simulink model "motor_bihuan_PI_tiaosu1205"  (Simulink 7.3)
settings: Solver=ode23tb  StartTime=0.0  StopTime=5  RelTol=1e-3
libraries: powerlib x12, powerlib_extras x2
settings Model: Creator=Administrator  LastModifiedBy=Administrator

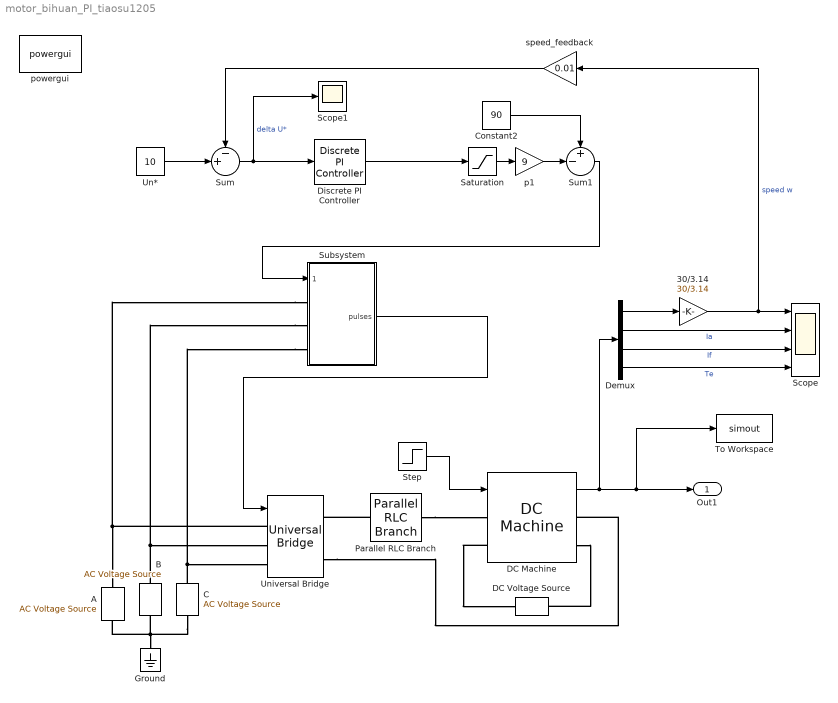
== system motor_bihuan_PI_tiaosu1205 ==
  30/3.14 : Gain  Gain=30/3.14  ParameterDataType=fixdt(1, 16)  ParameterScaling=2^0  OutDataType=fixdt(1, 16)  OutScaling=2^0
  A : powerlib/Electrical Sources/AC Voltage Source  DialogController=POWERSYS.PowerSysDialog  SystemSampleTime=-1  Amplitude=220  Phase=0  Frequency=50  SampleTime=0  Measurements=Voltage
  B : powerlib/Electrical Sources/AC Voltage Source  DialogController=POWERSYS.PowerSysDialog  SystemSampleTime=-1  Amplitude=220  Phase=240  Frequency=50  SampleTime=0  Measurements=Voltage
  C : powerlib/Electrical Sources/AC Voltage Source  DialogController=POWERSYS.PowerSysDialog  SystemSampleTime=-1  Amplitude=220  Phase=120  Frequency=50  SampleTime=0  Measurements=Voltage
  Constant2 : Constant  Value=90  OutDataType=fixdt(1, 16)  OutScaling=2^0
  DC Machine : powerlib/Machines/DC Machine  DialogController=POWERSYS.PowerSysDialog  SystemSampleTime=-1  PresetModel=No  MechanicalLoad=Torque TL  ShowDetailedParameters=on  RLa=[0.6 0.012]  RLf=[240 120]  Laf=1.8  J=1  Bm=0  Tf=0  w0=0  Ifinit=0.916666666666667  TsPowergui=0  TsBlock=-1
  DC Voltage Source : powerlib/Electrical Sources/DC Voltage Source  DialogController=POWERSYS.PowerSysDialog  SystemSampleTime=-1  Amplitude=220  Measurements=None
  Demux : Demux
  Discrete PI Controller : powerlib_extras/Discrete  Control Blocks/Discrete PI Controller  DialogController=POWERSYS.PowerSysDialog  SystemSampleTime=-1  Kp=1.2  Ki=2  Par_Limits=[1e6 -1e6]  Init=0  Ts=50e-6
  Ground : powerlib/Elements/Ground  DialogController=POWERSYS.PowerSysDialog  PhysicalDomain=powersysdomain  SubClassName=unknown  LeftPortType=p1  RightPortType=p1  LConnTagsString=a
  Parallel RLC Branch : powerlib/Elements/Parallel RLC Branch  DialogController=POWERSYS.PowerSysDialog  PhysicalDomain=powersysdomain  SubClassName=unknown  LeftPortType=p1  RightPortType=p1  LConnTagsString=a  RConnTagsString=__new0  BranchType=L  Resistance=1  Inductance=1e-3  SetiL0=off  InitialCurrent=0  Capacitance=1e-6  Setx0=off  InitialVoltage=0  Measurements=Branch voltage and current
  Saturation : Saturate  UpperLimit=10  LowerLimit=-10  OutDataType=fixdt(1, 16)  OutScaling=2^0
  Scope : Scope  NumInputPorts=4
      settings: TimeRange=5  YMin=-250~-50~0.870834~-100  YMax=1500~450~0.9625~800
  Scope1 : Scope
      settings: YMin=-0.5  YMax=1
  Step : Step  Time=2  Before=50  After=100  SampleTime=0
  Subsystem : Subsystem
  Sum : Sum  Inputs=-+|  OutDataType=fixdt(1, 16)  OutScaling=2^0
  Sum1 : Sum  Inputs=+-|  OutDataType=fixdt(1, 16)  OutScaling=2^0
  To Workspace : ToWorkspace  VariableName=simout  SampleTime=-1  SaveFormat=Structure
  Un* : Constant  Value=10  OutDataType=fixdt(1, 16)  OutScaling=2^0
  Universal Bridge : powerlib/Power Electronics/Universal Bridge  DialogController=POWERSYS.PowerSysDialog  SystemSampleTime=-1  Arms=3  SnubberResistance=1e5  SnubberCapacitance=inf  Device=Thyristors  Ron=1e-3  Lon=0  ForwardVoltages="[  0  0  ]"  ForwardVoltage=0  GTOparameters=[ 10e-6 , 20e-6 ]  IGBTparameters=[ 1e-6 , 2e-6 ]  Measurements=None  Measurements_2=None  converterType=Rectifier
  p1 : Gain  Gain=9  ParameterDataType=fixdt(1, 16)  ParameterScaling=2^0  OutDataType=fixdt(1, 16)  OutScaling=2^0
  powergui : powerlib/powergui  Priority=1  SystemSampleTime=-1  SimulationMode=Continuous  SampleTime=50e-6  frequency=60  SPID=off  DisableSnubberDevices=off  DisableRonSwitches=off  DisableVfSwitches=off  SwTol=0  Interpol=off  frequencyindice=0  echomessages=off  HookPort=off  DisplayEquations=off  FunctionMessages=off  EnableUseOfTLC=off  x0status=blocks  RestoreLinks=warning  Frange=[0:2:500]  Ylog=off  Xlog=on  ShowGrid=off  save=off  variable=ZData  ZoomFFT=on  StartTime=0.0  cycles=1  DisplayStyle=1  fundamental=60  FreqAxis=off  MaxFrequency=1000  frequencyindicesteady=1  RmsSteady=1  display=off  Ts=0  methode=off
  speed_feedback : Gain  Gain=0.01  ParameterDataType=fixdt(1, 16)  ParameterScaling=2^0  OutDataType=fixdt(1, 16)  OutScaling=2^0
  Out1 : Outport  OutDataType=fixdt(1, 16)  OutScaling=2^0
  wires:
  DC Machine/1 -> Demux/1, Out1/1, To Workspace/1
  Step/1 -> DC Machine/1
  Subsystem/1(pulses) -> Universal Bridge/1
  Demux/2 -> Scope/2  "Ia"
  Demux/3 -> Scope/3  "If"
  Demux/4 -> Scope/4  "Te"
  Demux/1 -> 30/3.14/1
  Un*/1 -> Sum/2
  30/3.14/1 -> Scope/1, speed_feedback/1  "speed w"
  speed_feedback/1 -> Sum/1
  Sum/1 -> Scope1/1, Discrete PI Controller/1  "delta U*"
  Saturation/1 -> p1/1
  p1/1 -> Sum1/2
  Constant2/1 -> Sum1/1
  Sum1/1 -> Subsystem/1(alpha_deg)
  Discrete PI Controller/1 -> Saturation/1
  connections:
  Parallel RLC Branch/LConn1 -- Universal Bridge/RConn1
  Parallel RLC Branch/RConn1 -- DC Machine/LConn1
  Universal Bridge/RConn2 -- DC Machine/RConn1
  DC Machine/LConn2 -- DC Voltage Source/RConn1
  DC Machine/RConn2 -- DC Voltage Source/LConn1
  C/LConn1 -- Ground/LConn1 -- B/LConn1 -- A/LConn1
  Subsystem/LConn1 -- Universal Bridge/LConn1 -- A/RConn1
  Subsystem/LConn2 -- B/RConn1 -- Universal Bridge/LConn2
  Subsystem/LConn3 -- C/RConn1 -- Universal Bridge/LConn3

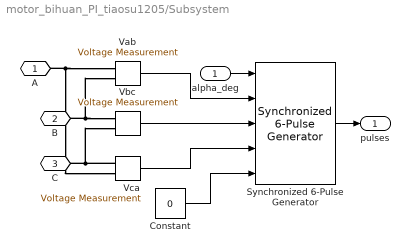
== system motor_bihuan_PI_tiaosu1205/Subsystem ==
  alpha_deg : Inport
  Constant : Constant  Value=0  OutDataType=fixdt(1, 16)  OutScaling=2^0
  Synchronized 6-Pulse Generator : powerlib_extras/Control  Blocks/Synchronized 6-Pulse Generator  DialogController=POWERSYS.PowerSysDialog  SystemSampleTime=-1  freq=50  pwidth=10  Double_Pulse=off
  Vab : powerlib/Measurements/Voltage Measurement  DialogController=POWERSYS.PowerSysDialog  SystemSampleTime=-1  PhasorSimulation=off  OutputType=Complex  PSBequivalent=0
  Vbc : powerlib/Measurements/Voltage Measurement  DialogController=POWERSYS.PowerSysDialog  SystemSampleTime=-1  PhasorSimulation=off  OutputType=Complex  PSBequivalent=0
  Vca : powerlib/Measurements/Voltage Measurement  DialogController=POWERSYS.PowerSysDialog  SystemSampleTime=-1  PhasorSimulation=off  OutputType=Complex  PSBequivalent=0
  A : PMIOPort  Port=1  Side=Left
  B : PMIOPort  Port=2  Side=Left
  C : PMIOPort  Port=3  Side=Left
  pulses : Outport
  wires:
  Vab/1 -> Synchronized 6-Pulse Generator/2
  Vbc/1 -> Synchronized 6-Pulse Generator/3
  Vca/1 -> Synchronized 6-Pulse Generator/4
  Constant/1 -> Synchronized 6-Pulse Generator/5
  alpha_deg/1 -> Synchronized 6-Pulse Generator/1
  Synchronized 6-Pulse Generator/1 -> pulses/1
  connections:
  A/RConn1 -- Vca/LConn2 -- Vab/LConn1
  B/RConn1 -- Vbc/LConn1 -- Vab/LConn2
  C/RConn1 -- Vca/LConn1 -- Vbc/LConn2
